simulink model "gm_uz_ssi_interface_2025b"  (R2025b)
settings: Solver=FixedStepDiscrete  StartTime=0.0  StopTime=0.005  RelTol=1e-3
undefined symbols (not defined in the file or in its folder): binary_or_gray, bit_sum, delay_first_clk_on_off, f_ADC, f_clock, PLL, ssi_clk_divider, ssi_encoder_bit_width_multi_turn, ssi_encoder_bit_width_single_turn, ssi_encoder_number_of_status_bits, t_ADC, t_clock, XData
libraries: hdlmdlgenlib x104, hdlsllib x90, simulink x33, simulink_extras x7
(part 4 of 4)

== system gm_uz_ssi_interface_2025b/uz_ssi_interface/position_to_speed_pll/Sine HDL Optimized1/sincos hdl ==
  In1 : Inport  OutDataTypeStr=fixdt(1, 27, 20)  SampleTime=1e-08
  cos_hdl : Subsystem  mask{NumDataPoints=double(256), TableDataTypeStr=fixdt(0,26,20), SimulateLUTROMDelay=Off}
      mask prompts: NumDataPoints "HDLShared:hdlshared:CosineHDL_Npts"; TableDataTypeStr "Simulink:blkprm_prompts:TABLE_UNIFIEDDATATYPE"; SimulateLUTROMDelay "HDLShared:hdlshared:CosineHDL_SimulateLUTDelay"
      mask init:
      | InputWordLength = double(10);
      | NumDataPoints = double(256);
      | OutputFracLength = double(20);
      | OutputWordLength = double(27);
      | SampleTime = double(-1);
      | SimulateLUTROMDelay = double(0);
      | TableDataTypeStr = fixdt(0,26,20);
      | TableFracLength = double(20);
      | TableWordLength = double(26);
      | YData = reshape(double([0;0.0061358846491544753;0.012271538285719925;0.01840672990580482;0.024541228522912288;0.030674803176636626;0.036807222941358832;0.04293825693494082;0.049067674327418015;0.055195244349689941;0.061320736302208578;0.067443919563664051;0.073564563599667426;0.079682437971430126;0.085797312344439894;0.091908956497132724;0.098017140329560604;0.10412163387205459;0.11022220729388306;0.11631863091190475;0.1224106751992162;0.12849811079379317;0.13458070850712617;0.14065823933284921;0.14673047445536175;0.15279718525844344;0.15885814333386145;0.16491312048996992;0.17096188876030122;0.17700422041214875;0.18303988795514095;0.18906866414980619;0.19509032201612825;0.2011046348420919;0.20711137619221856;0.21311031991609136;0.2191012401568698;0.22508391135979283;0.23105810828067111;0.2370236059943672;0.24298017990326387;0.24892760574572015;0.25486565960451457;0.26079411791527551;0.26671275747489837;0.27262135544994898;0.27851968938505306;0.28440753721127188;0.29028467725446233;0.29615088824362379;0.30200594931922808;0.30784964004153487;0.31368174039889152;0.31950203081601569;0.32531029216226293;0.33110630575987643;0.33688985339222005;0.34266071731199438;0.34841868024943456;0.35416352542049034;0.35989503653498811;0.36561299780477385;0.37131719395183749;0.37700741021641826;0.38268343236508978;0.38834504669882625;0.3939920400610481;0.39962419984564679;0.40524131400498986;0.41084317105790391;0.41642956009763715;0.42200027079979968;0.42755509343028208;0.43309381885315196;0.43861623853852766;0.4441221445704292;0.44961132965460654;0.45508358712634384;0.46053871095824001;0.46597649576796618;0.47139673682599764;0.47679923006332209;0.48218377207912272;0.487550160148436;0.49289819222978404;0.49822766697278181;0.50353838372571758;0.50883014254310699;0.51410274419322166;0.51935599016558964;0.52458968267846895;0.52980362468629461;0.53499761988709715;0.54017147272989285;0.54532498842204646;0.55045797293660481;0.55557023301960218;0.56066157619733603;0.56573181078361312;0.57078074588696726;0.57580819141784534;0.58081395809576453;0.58579785745643886;0.59075970185887416;0.59569930449243336;0.60061647938386897;0.60551104140432555;0.61038280627630948;0.61523159058062682;0.6200572117632891;0.62485948814238634;0.62963823891492698;0.63439328416364549;0.63912444486377573;0.64383154288979139;0.64851440102211244;0.65317284295377676;0.65780669329707864;0.66241577759017178;0.66699992230363747;0.67155895484701833;0.67609270357531592;0.68060099779545302;0.68508366777270036;0.68954054473706683;0.69397146088965389;0.69837624940897292;0.7027547444572253;0.70710678118654746;0.71143219574521643;0.71573082528381859;0.72000250796138165;0.72424708295146689;0.7284643904482252;0.73265427167241282;0.73681656887736979;0.74095112535495911;0.74505778544146595;0.74913639452345926;0.75318679904361252;0.75720884650648457;0.76120238548426178;0.76516726562245896;0.76910333764557959;0.77301045336273688;0.77688846567323244;0.78073722857209438;0.78455659715557524;0.78834642762660623;0.79210657730021228;0.79583690460888357;0.79953726910790501;0.80320753148064483;0.80684755354379922;0.81045719825259477;0.8140363297059483;0.81758481315158371;0.82110251499110465;0.82458930278502529;0.8280450452577558;0.83146961230254524;0.83486287498638001;0.83822470555483797;0.84155497743689833;0.84485356524970701;0.84812034480329712;0.8513551931052652;0.85455798836540053;0.85772861000027212;0.86086693863776731;0.8639728561215867;0.86704624551569265;0.87008699110871135;0.87309497841829009;0.8760700941954066;0.87901222642863341;0.88192126434835494;0.88479709843093779;0.88763962040285393;0.89044872324475788;0.89322430119551532;0.89596624975618511;0.89867446569395382;0.90134884704602203;0.90398929312344334;0.90659570451491533;0.90916798309052238;0.91170603200542988;0.91420975570353069;0.9166790599210427;0.91911385169005777;0.9215140393420419;0.92387953251128674;0.92621024213831138;0.92850608047321559;0.93076696107898371;0.93299279883473885;0.9351835099389475;0.93733901191257496;0.93945922360218992;0.94154406518302081;0.94359345816196039;0.94560732538052128;0.94758559101774109;0.94952818059303667;0.95143502096900834;0.95330604035419375;0.95514116830577067;0.95694033573220894;0.9587034748958716;0.96043051941556579;0.96212140426904158;0.96377606579543984;0.9653944416976894;0.96697647104485207;0.96852209427441727;0.97003125319454397;0.97150389098625178;0.97293995220556007;0.97433938278557586;0.97570213003852857;0.97702814265775439;0.97831737071962765;0.97956976568544052;0.98078528040323043;0.98196386910955524;0.98310548743121629;0.98421009238692903;0.98527764238894122;0.98630809724459867;0.98730141815785843;0.98825756773074946;0.98917650996478101;0.99005821026229712;0.99090263542778001;0.99170975366909953;0.99247953459870997;0.9932119492347945;0.99390697000235606;0.99456457073425542;0.99518472667219682;0.99576741446765982;0.996312612182778;0.99682029929116567;0.99729045667869021;0.99772306664419164;0.99811811290014918;0.99847558057329477;0.99879545620517241;0.99907772775264536;0.99932238458834954;0.99952941750109314;0.99969881869620425;0.9998305817958234;0.9999247018391445;0.99998117528260111]), [1  256]);
      | block_name = 'uz_ssi_interface_2025b/uz_ssi_interface/position_to_speed_pll/Sine\nHDL Optimized1/sincos hdl/cos_hdl';
      | gcb_lut = double(11088.000122070312);
      mask Display:
      | port_label('input',1,'u')
      | port_label('output',1,'cos(2*pi*u)')
      | xpos = 0.35;
      | yoffset = 0.5;
      | if ( SimulateLUTROMDelay )
      |   text(xpos,yoffset,'HDL (Z^{-1})','texmode','on')
      | else
      |    text(xpos,yoffset,'HDL')
      | end
  sin_hdl : Subsystem  mask{NumDataPoints=double(256), TableDataTypeStr=fixdt(0,26,20), SimulateLUTROMDelay=Off}
      mask prompts: NumDataPoints "HDLShared:hdlshared:CosineHDL_Npts"; TableDataTypeStr "Simulink:blkprm_prompts:TABLE_UNIFIEDDATATYPE"; SimulateLUTROMDelay "HDLShared:hdlshared:CosineHDL_SimulateLUTDelay"
      mask init:
      | InputWordLength = double(10);
      | NumDataPoints = double(256);
      | OutputFracLength = double(20);
      | OutputWordLength = double(27);
      | SampleTime = double(-1);
      | SimulateLUTROMDelay = double(0);
      | TableDataTypeStr = fixdt(0,26,20);
      | TableFracLength = double(20);
      | TableWordLength = double(26);
      | YData = reshape(double([0;0.0061358846491544753;0.012271538285719925;0.01840672990580482;0.024541228522912288;0.030674803176636626;0.036807222941358832;0.04293825693494082;0.049067674327418015;0.055195244349689941;0.061320736302208578;0.067443919563664051;0.073564563599667426;0.079682437971430126;0.085797312344439894;0.091908956497132724;0.098017140329560604;0.10412163387205459;0.11022220729388306;0.11631863091190475;0.1224106751992162;0.12849811079379317;0.13458070850712617;0.14065823933284921;0.14673047445536175;0.15279718525844344;0.15885814333386145;0.16491312048996992;0.17096188876030122;0.17700422041214875;0.18303988795514095;0.18906866414980619;0.19509032201612825;0.2011046348420919;0.20711137619221856;0.21311031991609136;0.2191012401568698;0.22508391135979283;0.23105810828067111;0.2370236059943672;0.24298017990326387;0.24892760574572015;0.25486565960451457;0.26079411791527551;0.26671275747489837;0.27262135544994898;0.27851968938505306;0.28440753721127188;0.29028467725446233;0.29615088824362379;0.30200594931922808;0.30784964004153487;0.31368174039889152;0.31950203081601569;0.32531029216226293;0.33110630575987643;0.33688985339222005;0.34266071731199438;0.34841868024943456;0.35416352542049034;0.35989503653498811;0.36561299780477385;0.37131719395183749;0.37700741021641826;0.38268343236508978;0.38834504669882625;0.3939920400610481;0.39962419984564679;0.40524131400498986;0.41084317105790391;0.41642956009763715;0.42200027079979968;0.42755509343028208;0.43309381885315196;0.43861623853852766;0.4441221445704292;0.44961132965460654;0.45508358712634384;0.46053871095824001;0.46597649576796618;0.47139673682599764;0.47679923006332209;0.48218377207912272;0.487550160148436;0.49289819222978404;0.49822766697278181;0.50353838372571758;0.50883014254310699;0.51410274419322166;0.51935599016558964;0.52458968267846895;0.52980362468629461;0.53499761988709715;0.54017147272989285;0.54532498842204646;0.55045797293660481;0.55557023301960218;0.56066157619733603;0.56573181078361312;0.57078074588696726;0.57580819141784534;0.58081395809576453;0.58579785745643886;0.59075970185887416;0.59569930449243336;0.60061647938386897;0.60551104140432555;0.61038280627630948;0.61523159058062682;0.6200572117632891;0.62485948814238634;0.62963823891492698;0.63439328416364549;0.63912444486377573;0.64383154288979139;0.64851440102211244;0.65317284295377676;0.65780669329707864;0.66241577759017178;0.66699992230363747;0.67155895484701833;0.67609270357531592;0.68060099779545302;0.68508366777270036;0.68954054473706683;0.69397146088965389;0.69837624940897292;0.7027547444572253;0.70710678118654746;0.71143219574521643;0.71573082528381859;0.72000250796138165;0.72424708295146689;0.7284643904482252;0.73265427167241282;0.73681656887736979;0.74095112535495911;0.74505778544146595;0.74913639452345926;0.75318679904361252;0.75720884650648457;0.76120238548426178;0.76516726562245896;0.76910333764557959;0.77301045336273688;0.77688846567323244;0.78073722857209438;0.78455659715557524;0.78834642762660623;0.79210657730021228;0.79583690460888357;0.79953726910790501;0.80320753148064483;0.80684755354379922;0.81045719825259477;0.8140363297059483;0.81758481315158371;0.82110251499110465;0.82458930278502529;0.8280450452577558;0.83146961230254524;0.83486287498638001;0.83822470555483797;0.84155497743689833;0.84485356524970701;0.84812034480329712;0.8513551931052652;0.85455798836540053;0.85772861000027212;0.86086693863776731;0.8639728561215867;0.86704624551569265;0.87008699110871135;0.87309497841829009;0.8760700941954066;0.87901222642863341;0.88192126434835494;0.88479709843093779;0.88763962040285393;0.89044872324475788;0.89322430119551532;0.89596624975618511;0.89867446569395382;0.90134884704602203;0.90398929312344334;0.90659570451491533;0.90916798309052238;0.91170603200542988;0.91420975570353069;0.9166790599210427;0.91911385169005777;0.9215140393420419;0.92387953251128674;0.92621024213831138;0.92850608047321559;0.93076696107898371;0.93299279883473885;0.9351835099389475;0.93733901191257496;0.93945922360218992;0.94154406518302081;0.94359345816196039;0.94560732538052128;0.94758559101774109;0.94952818059303667;0.95143502096900834;0.95330604035419375;0.95514116830577067;0.95694033573220894;0.9587034748958716;0.96043051941556579;0.96212140426904158;0.96377606579543984;0.9653944416976894;0.96697647104485207;0.96852209427441727;0.97003125319454397;0.97150389098625178;0.97293995220556007;0.97433938278557586;0.97570213003852857;0.97702814265775439;0.97831737071962765;0.97956976568544052;0.98078528040323043;0.98196386910955524;0.98310548743121629;0.98421009238692903;0.98527764238894122;0.98630809724459867;0.98730141815785843;0.98825756773074946;0.98917650996478101;0.99005821026229712;0.99090263542778001;0.99170975366909953;0.99247953459870997;0.9932119492347945;0.99390697000235606;0.99456457073425542;0.99518472667219682;0.99576741446765982;0.996312612182778;0.99682029929116567;0.99729045667869021;0.99772306664419164;0.99811811290014918;0.99847558057329477;0.99879545620517241;0.99907772775264536;0.99932238458834954;0.99952941750109314;0.99969881869620425;0.9998305817958234;0.9999247018391445;0.99998117528260111]), [1  256]);
      | block_name = 'uz_ssi_interface_2025b/uz_ssi_interface/position_to_speed_pll/Sine\nHDL Optimized1/sincos hdl/sin_hdl';
      | gcb_lut = double(11232.000122070312);
      mask Display:
      | port_label('input',1,'u')
      | port_label('output',1,'sin(2*pi*u)')
      | xpos = 0.35;
      | yoffset = 0.5;
      | if ( SimulateLUTROMDelay )
      |   text(xpos,yoffset,'HDL (Z^{-1})','texmode','on')
      | else
      |    text(xpos,yoffset,'HDL')
      | end
  Out1 : Outport  SampleTime=1e-08  VectorParamsAs1DForOutWhenUnconnected=off
  Out2 : Outport  Port=2  SampleTime=1e-08  VectorParamsAs1DForOutWhenUnconnected=off
  wires:
  In1/1 -> cos_hdl/1(In1), sin_hdl/1(In1)
  sin_hdl/1(y) -> Out1/1
  cos_hdl/1(x) -> Out2/1

== system gm_uz_ssi_interface_2025b/uz_ssi_interface/ssi_communication/sample_serial_ssi_data/Sample and Hold1 ==
  In : Inport  OutDataTypeStr=boolean  SampleTime=1e-08
  S : Inport  Port=2  OutDataTypeStr=boolean  SampleTime=1e-08
  Model : Subsystem
  "   " : Outport  SampleTime=1e-08  InitialOutput=0  VectorParamsAs1DForOutWhenUnconnected=off
  wires:
  In/1 -> Model/1(In)
  S/1 -> Model/2(S)
  Model/1(Out) -> "   "/1

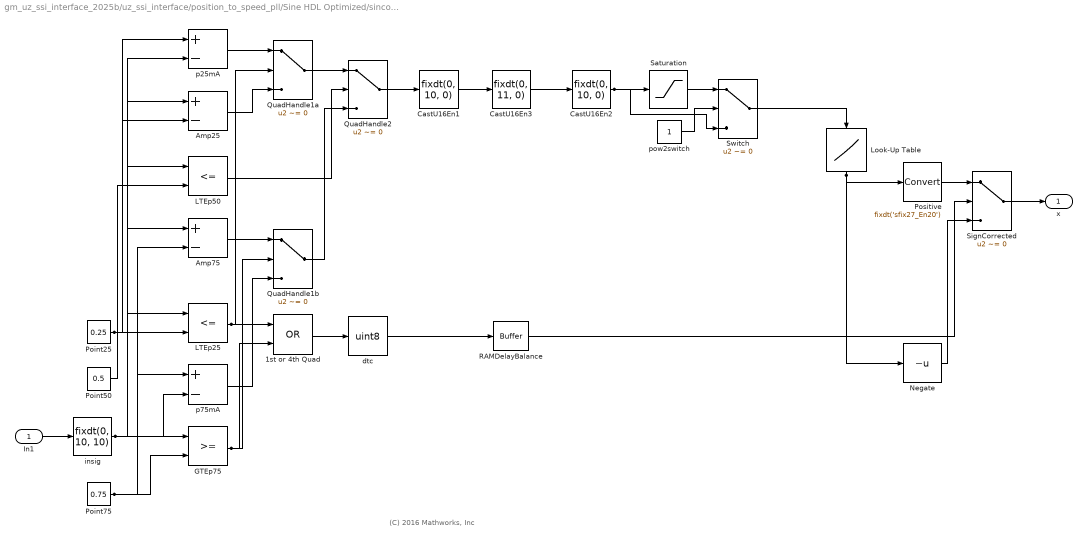
== system gm_uz_ssi_interface_2025b/uz_ssi_interface/position_to_speed_pll/Sine HDL Optimized/sincos hdl/cos_hdl ==
  note: (C) 2016 Mathworks, Inc
  In1 : Inport  OutDataTypeStr=fixdt(1, 27, 20)  SampleTime=1e-08
  1st or 4th Quad : Logic  Operator=OR  AllPortsSameDT=off  OutDataTypeStr=boolean  SampleTime=1e-08
  Amp25 : Sum  Inputs=+-  OutDataTypeStr=fixdt(1, 28, 27)  AccumDataTypeStr=fixdt(1, 28, 27)  SampleTime=1e-08
  Amp75 : Sum  Inputs=+-  OutDataTypeStr=fixdt(1, 28, 27)  AccumDataTypeStr=fixdt(1, 28, 27)  SampleTime=1e-08
  CastU16En1 : DataTypeConversion  OutDataTypeStr=fixdt(0, 10, 0)  ConvertRealWorld=Stored Integer (SI)  SampleTime=1e-08  SaturateOnIntegerOverflow=off  RndMeth=Floor
  CastU16En2 : DataTypeConversion  OutDataTypeStr=fixdt(0, 10, 0)  ConvertRealWorld=Stored Integer (SI)  SampleTime=1e-08  RndMeth=Floor
  CastU16En3 : DataTypeConversion  OutDataTypeStr=fixdt(0, 11, 0)  SampleTime=1e-08  SaturateOnIntegerOverflow=off  RndMeth=Floor
  GTEp75 : RelationalOperator  OutDataTypeStr=boolean  SampleTime=1e-08  InputSameDT=off
  LTEp25 : RelationalOperator  Operator=<=  OutDataTypeStr=boolean  SampleTime=1e-08  InputSameDT=off
  LTEp50 : RelationalOperator  Operator=<=  OutDataTypeStr=boolean  SampleTime=1e-08  InputSameDT=off
  Look-Up Table : Lookup_n-D  NumberOfTableDimensions=1  LookupTableObject=''  BreakpointsSpecification=Even spacing  BreakpointsForDimension1=XData  BreakpointsForDimension1FirstPoint=fi(0,0,InputWordLength,0)  BreakpointsForDimension1Spacing=fi(1,0,InputWordLength,0)  IndexSearchMethod=Evenly spaced points  Table=fi(YData,0, TableWordLength, TableFracLength)  TableDataTypeStr=fixdt(0, TableWordLength, TableFracLength)  InterpMethod=Flat  ExtrapMethod=Clip  OutDataTypeStr=fixdt(1,OutputWordLength,OutputFracLength)  LockScale=on
  Negate : UnaryMinus  SampleTime=1e-08
  Point25 : Constant  Value=0.25  OutDataTypeStr=fixdt(0, 27, 27)  SampleTime=1e-08
  Point50 : Constant  Value=0.5  OutDataTypeStr=fixdt(0, 27, 27)  SampleTime=1e-08
  Point75 : Constant  Value=0.75  OutDataTypeStr=fixdt(0, 27, 27)  SampleTime=1e-08
  Positive : DataTypeConversion  OutDataTypeStr=fixdt('sfix27_En20')
  QuadHandle1a : Switch  Criteria=u2 ~= 0  Threshold="fi(0,0,1,0,\"hex\",\"0\")"  OutDataTypeStr=fixdt(1, 28, 27)  SampleTime=1e-08  SaturateOnIntegerOverflow=off  InputSameDT=off
  QuadHandle1b : Switch  Criteria=u2 ~= 0  Threshold="fi(0,0,1,0,\"hex\",\"0\")"  OutDataTypeStr=fixdt(1, 28, 27)  SampleTime=1e-08  SaturateOnIntegerOverflow=off  InputSameDT=off
  QuadHandle2 : Switch  Criteria=u2 ~= 0  Threshold="fi(0,0,1,0,\"hex\",\"0\")"  OutDataTypeStr=fixdt(0, 10, 10)  SampleTime=1e-08  InputSameDT=off
  RAMDelayBalance : hdlmdlgenlib/Buffer
  Saturation : Saturate  UpperLimit="fi(0,0,10,0,\"hex\",\"0ff\")"  LowerLimit="fi(0,0,10,0,\"hex\",\"000\")"  SampleTime=1e-08  OutDataTypeStr=fixdt(0, 10, 0)
  SignCorrected : Switch  Criteria=u2 ~= 0  Threshold="fi(0,0,8,0,\"hex\",\"00\")"  OutDataTypeStr=fixdt(1, 27, 20)  SampleTime=1e-08  SaturateOnIntegerOverflow=off  InputSameDT=off
  Switch : Switch  Criteria=u2 ~= 0  Threshold="fi(0,0,1,0,\"hex\",\"0\")"  OutDataTypeStr=fixdt(0, 10, 0)  SampleTime=1e-08  SaturateOnIntegerOverflow=off  InputSameDT=off
  dtc : DataTypeConversion  OutDataTypeStr=uint8  ConvertRealWorld=Stored Integer (SI)  SampleTime=1e-08  SaturateOnIntegerOverflow=off  RndMeth=Floor
  insig : DataTypeConversion  OutDataTypeStr=fixdt(0, 10, 10)  SampleTime=1e-08  SaturateOnIntegerOverflow=off  RndMeth=Floor
  p25mA : Sum  Inputs=+-  OutDataTypeStr=fixdt(1, 28, 27)  AccumDataTypeStr=fixdt(1, 28, 27)  SampleTime=1e-08
  p75mA : Sum  Inputs=+-  OutDataTypeStr=fixdt(1, 28, 27)  AccumDataTypeStr=fixdt(1, 28, 27)  SampleTime=1e-08
  pow2switch : Constant  OutDataTypeStr=boolean  SampleTime=1e-08
  x : Outport  SampleTime=1e-08  VectorParamsAs1DForOutWhenUnconnected=off
  wires:
  In1/1 -> insig/1
  p25mA/1 -> QuadHandle1a/1
  Point25/1 -> p25mA/1, LTEp25/2, Amp25/2
  Point50/1 -> LTEp50/2
  Amp25/1 -> QuadHandle1a/3
  insig/1 -> p25mA/2, LTEp50/1, LTEp25/1, GTEp75/1, Amp75/1, p75mA/2, Amp25/1
  Point75/1 -> GTEp75/2, p75mA/1, Amp75/2
  LTEp50/1 -> QuadHandle2/2
  Amp75/1 -> QuadHandle1b/1
  LTEp25/1 -> QuadHandle1a/2, 1st or 4th Quad/1
  p75mA/1 -> QuadHandle1b/3
  GTEp75/1 -> QuadHandle1b/2, 1st or 4th Quad/2
  QuadHandle1a/1 -> QuadHandle2/1
  QuadHandle1b/1 -> QuadHandle2/3
  1st or 4th Quad/1 -> dtc/1
  Saturation/1 -> Switch/1
  QuadHandle2/1 -> CastU16En1/1
  dtc/1 -> RAMDelayBalance/1
  CastU16En1/1 -> CastU16En3/1
  CastU16En2/1 -> Switch/3, Saturation/1
  CastU16En3/1 -> CastU16En2/1
  RAMDelayBalance/1 -> SignCorrected/2
  SignCorrected/1 -> x/1
  pow2switch/1 -> Switch/2
  Switch/1 -> Look-Up Table/1
  Look-Up Table/1 -> Positive/1, Negate/1
  Positive/1 -> SignCorrected/1
  Negate/1 -> SignCorrected/3

== system gm_uz_ssi_interface_2025b/uz_ssi_interface/position_to_speed_pll/Sine HDL Optimized/sincos hdl/sin_hdl ==
  note: (C) 2016 Mathworks, Inc
  In1 : Inport  OutDataTypeStr=fixdt(1, 27, 20)  SampleTime=1e-08
  Amp50 : Sum  Inputs=+-  OutDataTypeStr=fixdt(1, 28, 27)  AccumDataTypeStr=fixdt(1, 28, 27)  SampleTime=1e-08
  CastU16En2 : DataTypeConversion  OutDataTypeStr=fixdt(0, 10, 0)  ConvertRealWorld=Stored Integer (SI)  SampleTime=1e-08  SaturateOnIntegerOverflow=off  RndMeth=Floor
  CastU16En3 : DataTypeConversion  OutDataTypeStr=fixdt(0, 10, 0)  ConvertRealWorld=Stored Integer (SI)  SampleTime=1e-08  RndMeth=Floor
  CastU16En4 : DataTypeConversion  OutDataTypeStr=fixdt(0, 11, 0)  SampleTime=1e-08  SaturateOnIntegerOverflow=off  RndMeth=Floor
  LTEp25 : RelationalOperator  Operator=<=  OutDataTypeStr=boolean  SampleTime=1e-08  InputSameDT=off
  LTEp50 : RelationalOperator  Operator=<=  OutDataTypeStr=boolean  SampleTime=1e-08  InputSameDT=off
  Look-Up Table : Lookup_n-D  NumberOfTableDimensions=1  LookupTableObject=''  BreakpointsSpecification=Even spacing  BreakpointsForDimension1=XData  BreakpointsForDimension1FirstPoint=fi(0,0,InputWordLength,0)  BreakpointsForDimension1Spacing=fi(1,0,InputWordLength,0)  IndexSearchMethod=Evenly spaced points  Table=fi(YData,0, TableWordLength, TableFracLength)  TableDataTypeStr=fixdt(0, TableWordLength, TableFracLength)  InterpMethod=Flat  ExtrapMethod=Clip  OutDataTypeStr=fixdt(1,OutputWordLength,OutputFracLength)  LockScale=on
  Negate : UnaryMinus  SampleTime=1e-08
  Point25 : Constant  Value=0.25  OutDataTypeStr=fixdt(0, 27, 27)  SampleTime=1e-08
  Point50 : Constant  Value=0.5  OutDataTypeStr=fixdt(0, 27, 27)  SampleTime=1e-08
  Positive : DataTypeConversion  OutDataTypeStr=fixdt('sfix27_En20')
  QuadHandle1 : Switch  Criteria=u2 ~= 0  Threshold="fi(0,0,1,0,\"hex\",\"0\")"  OutDataTypeStr=fixdt(1, 28, 27)  SampleTime=1e-08  SaturateOnIntegerOverflow=off  InputSameDT=off
  QuadHandle2 : Switch  Criteria=u2 ~= 0  Threshold="fi(0,0,1,0,\"hex\",\"0\")"  OutDataTypeStr=fixdt(0, 10, 10)  SampleTime=1e-08  SaturateOnIntegerOverflow=off  InputSameDT=off
  RAMDelayBalance : hdlmdlgenlib/Buffer
  Saturation : Saturate  UpperLimit="fi(0,0,10,0,\"hex\",\"0ff\")"  LowerLimit="fi(0,0,10,0,\"hex\",\"000\")"  SampleTime=1e-08  OutDataTypeStr=fixdt(0, 10, 0)
  SignCorrected : Switch  Criteria=u2 ~= 0  Threshold="fi(0,0,1,0,\"hex\",\"0\")"  OutDataTypeStr=fixdt(1, 27, 20)  SampleTime=1e-08  SaturateOnIntegerOverflow=off  InputSameDT=off
  Switch : Switch  Criteria=u2 ~= 0  Threshold="fi(0,0,1,0,\"hex\",\"0\")"  OutDataTypeStr=fixdt(0, 10, 0)  SampleTime=1e-08  SaturateOnIntegerOverflow=off  InputSameDT=off
  insig : DataTypeConversion  OutDataTypeStr=fixdt(0, 10, 10)  SampleTime=1e-08  SaturateOnIntegerOverflow=off  RndMeth=Floor
  p50mA : Sum  Inputs=+-  OutDataTypeStr=fixdt(1, 29, 27)  AccumDataTypeStr=fixdt(1, 29, 27)  SampleTime=1e-08
  pow2switch : Constant  OutDataTypeStr=boolean  SampleTime=1e-08
  y : Outport  SampleTime=1e-08  VectorParamsAs1DForOutWhenUnconnected=off
  wires:
  LTEp25/1 -> QuadHandle2/2
  Negate/1 -> SignCorrected/3
  QuadHandle1/1 -> QuadHandle2/1, p50mA/2, LTEp25/1
  Point50/1 -> p50mA/1, LTEp50/2, Amp50/2
  In1/1 -> insig/1
  Switch/1 -> Look-Up Table/1
  insig/1 -> QuadHandle1/1, LTEp50/1, Amp50/1
  Amp50/1 -> QuadHandle1/3
  LTEp50/1 -> RAMDelayBalance/1, QuadHandle1/2
  Point25/1 -> LTEp25/2
  p50mA/1 -> QuadHandle2/3
  RAMDelayBalance/1 -> SignCorrected/2
  QuadHandle2/1 -> CastU16En2/1
  CastU16En3/1 -> Switch/3, Saturation/1
  CastU16En2/1 -> CastU16En4/1
  CastU16En4/1 -> CastU16En3/1
  Saturation/1 -> Switch/1
  pow2switch/1 -> Switch/2
  Look-Up Table/1 -> Positive/1, Negate/1
  Positive/1 -> SignCorrected/1
  SignCorrected/1 -> y/1

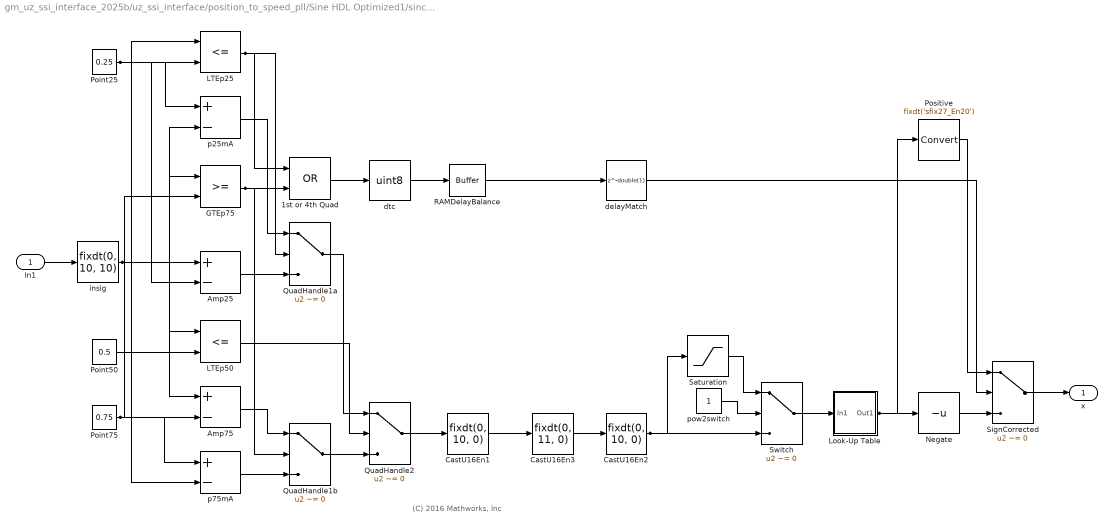
== system gm_uz_ssi_interface_2025b/uz_ssi_interface/position_to_speed_pll/Sine HDL Optimized1/sincos hdl/cos_hdl ==
  note: (C) 2016 Mathworks, Inc
  In1 : Inport  OutDataTypeStr=fixdt(1, 27, 20)  SampleTime=1e-08
  1st or 4th Quad : Logic  Operator=OR  AllPortsSameDT=off  OutDataTypeStr=boolean  SampleTime=1e-08
  Amp25 : Sum  Inputs=+-  OutDataTypeStr=fixdt(1, 28, 27)  AccumDataTypeStr=fixdt(1, 28, 27)  SampleTime=1e-08
  Amp75 : Sum  Inputs=+-  OutDataTypeStr=fixdt(1, 28, 27)  AccumDataTypeStr=fixdt(1, 28, 27)  SampleTime=1e-08
  CastU16En1 : DataTypeConversion  OutDataTypeStr=fixdt(0, 10, 0)  ConvertRealWorld=Stored Integer (SI)  SampleTime=1e-08  SaturateOnIntegerOverflow=off  RndMeth=Floor
  CastU16En2 : DataTypeConversion  OutDataTypeStr=fixdt(0, 10, 0)  ConvertRealWorld=Stored Integer (SI)  SampleTime=1e-08  RndMeth=Floor
  CastU16En3 : DataTypeConversion  OutDataTypeStr=fixdt(0, 11, 0)  SampleTime=1e-08  SaturateOnIntegerOverflow=off  RndMeth=Floor
  GTEp75 : RelationalOperator  OutDataTypeStr=boolean  SampleTime=1e-08  InputSameDT=off
  LTEp25 : RelationalOperator  Operator=<=  OutDataTypeStr=boolean  SampleTime=1e-08  InputSameDT=off
  LTEp50 : RelationalOperator  Operator=<=  OutDataTypeStr=boolean  SampleTime=1e-08  InputSameDT=off
  Look-Up Table : Subsystem
  Negate : UnaryMinus  SampleTime=1e-08
  Point25 : Constant  Value=0.25  OutDataTypeStr=fixdt(0, 27, 27)  SampleTime=1e-08
  Point50 : Constant  Value=0.5  OutDataTypeStr=fixdt(0, 27, 27)  SampleTime=1e-08
  Point75 : Constant  Value=0.75  OutDataTypeStr=fixdt(0, 27, 27)  SampleTime=1e-08
  Positive : DataTypeConversion  OutDataTypeStr=fixdt('sfix27_En20')
  QuadHandle1a : Switch  Criteria=u2 ~= 0  Threshold="fi(0,0,1,0,\"hex\",\"0\")"  OutDataTypeStr=fixdt(1, 28, 27)  SampleTime=1e-08  SaturateOnIntegerOverflow=off  InputSameDT=off
  QuadHandle1b : Switch  Criteria=u2 ~= 0  Threshold="fi(0,0,1,0,\"hex\",\"0\")"  OutDataTypeStr=fixdt(1, 28, 27)  SampleTime=1e-08  SaturateOnIntegerOverflow=off  InputSameDT=off
  QuadHandle2 : Switch  Criteria=u2 ~= 0  Threshold="fi(0,0,1,0,\"hex\",\"0\")"  OutDataTypeStr=fixdt(0, 10, 10)  SampleTime=1e-08  InputSameDT=off
  RAMDelayBalance : hdlmdlgenlib/Buffer
  Saturation : Saturate  UpperLimit="fi(0,0,10,0,\"hex\",\"0ff\")"  LowerLimit="fi(0,0,10,0,\"hex\",\"000\")"  SampleTime=1e-08  OutDataTypeStr=fixdt(0, 10, 0)
  SignCorrected : Switch  Criteria=u2 ~= 0  Threshold="fi(0,0,8,0,\"hex\",\"00\")"  OutDataTypeStr=fixdt(1, 27, 20)  SampleTime=1e-08  SaturateOnIntegerOverflow=off  InputSameDT=off
  Switch : Switch  Criteria=u2 ~= 0  Threshold="fi(0,0,1,0,\"hex\",\"0\")"  OutDataTypeStr=fixdt(0, 10, 0)  SampleTime=1e-08  SaturateOnIntegerOverflow=off  InputSameDT=off
  delayMatch : Delay  DelayLength=double(1)  InitialCondition=0
  dtc : DataTypeConversion  OutDataTypeStr=uint8  ConvertRealWorld=Stored Integer (SI)  SampleTime=1e-08  SaturateOnIntegerOverflow=off  RndMeth=Floor
  insig : DataTypeConversion  OutDataTypeStr=fixdt(0, 10, 10)  SampleTime=1e-08  SaturateOnIntegerOverflow=off  RndMeth=Floor
  p25mA : Sum  Inputs=+-  OutDataTypeStr=fixdt(1, 28, 27)  AccumDataTypeStr=fixdt(1, 28, 27)  SampleTime=1e-08
  p75mA : Sum  Inputs=+-  OutDataTypeStr=fixdt(1, 28, 27)  AccumDataTypeStr=fixdt(1, 28, 27)  SampleTime=1e-08
  pow2switch : Constant  OutDataTypeStr=boolean  SampleTime=1e-08
  x : Outport  SampleTime=1e-08  VectorParamsAs1DForOutWhenUnconnected=off
  wires:
  GTEp75/1 -> QuadHandle1b/2, 1st or 4th Quad/2
  In1/1 -> insig/1
  delayMatch/1 -> SignCorrected/2
  Point25/1 -> p25mA/1, LTEp25/2, Amp25/2
  Point50/1 -> LTEp50/2
  insig/1 -> p25mA/2, LTEp25/1, GTEp75/1, p75mA/2, Amp75/1, Amp25/1, LTEp50/1
  pow2switch/1 -> Switch/2
  QuadHandle1a/1 -> QuadHandle2/1
  Point75/1 -> GTEp75/2, Amp75/2, p75mA/1
  LTEp25/1 -> 1st or 4th Quad/1, QuadHandle1a/2
  p25mA/1 -> QuadHandle1a/1
  Amp25/1 -> QuadHandle1a/3
  LTEp50/1 -> QuadHandle2/2
  CastU16En1/1 -> CastU16En3/1
  Amp75/1 -> QuadHandle1b/1
  p75mA/1 -> QuadHandle1b/3
  1st or 4th Quad/1 -> dtc/1
  QuadHandle1b/1 -> QuadHandle2/3
  dtc/1 -> RAMDelayBalance/1
  QuadHandle2/1 -> CastU16En1/1
  RAMDelayBalance/1 -> delayMatch/1
  CastU16En3/1 -> CastU16En2/1
  CastU16En2/1 -> Switch/3, Saturation/1
  Saturation/1 -> Switch/1
  Switch/1 -> Look-Up Table/1(In1)
  Look-Up Table/1(Out1) -> Negate/1, Positive/1
  Negate/1 -> SignCorrected/3
  Positive/1 -> SignCorrected/1
  SignCorrected/1 -> x/1

== system gm_uz_ssi_interface_2025b/uz_ssi_interface/position_to_speed_pll/Sine HDL Optimized1/sincos hdl/sin_hdl ==
  note: (C) 2016 Mathworks, Inc
  In1 : Inport  OutDataTypeStr=fixdt(1, 27, 20)  SampleTime=1e-08
  Amp50 : Sum  Inputs=+-  OutDataTypeStr=fixdt(1, 28, 27)  AccumDataTypeStr=fixdt(1, 28, 27)  SampleTime=1e-08
  CastU16En2 : DataTypeConversion  OutDataTypeStr=fixdt(0, 10, 0)  ConvertRealWorld=Stored Integer (SI)  SampleTime=1e-08  SaturateOnIntegerOverflow=off  RndMeth=Floor
  CastU16En3 : DataTypeConversion  OutDataTypeStr=fixdt(0, 10, 0)  ConvertRealWorld=Stored Integer (SI)  SampleTime=1e-08  RndMeth=Floor
  CastU16En4 : DataTypeConversion  OutDataTypeStr=fixdt(0, 11, 0)  SampleTime=1e-08  SaturateOnIntegerOverflow=off  RndMeth=Floor
  LTEp25 : RelationalOperator  Operator=<=  OutDataTypeStr=boolean  SampleTime=1e-08  InputSameDT=off
  LTEp50 : RelationalOperator  Operator=<=  OutDataTypeStr=boolean  SampleTime=1e-08  InputSameDT=off
  Look-Up Table : Subsystem
  Negate : UnaryMinus  SampleTime=1e-08
  Point25 : Constant  Value=0.25  OutDataTypeStr=fixdt(0, 27, 27)  SampleTime=1e-08
  Point50 : Constant  Value=0.5  OutDataTypeStr=fixdt(0, 27, 27)  SampleTime=1e-08
  Positive : DataTypeConversion  OutDataTypeStr=fixdt('sfix27_En20')
  QuadHandle1 : Switch  Criteria=u2 ~= 0  Threshold="fi(0,0,1,0,\"hex\",\"0\")"  OutDataTypeStr=fixdt(1, 28, 27)  SampleTime=1e-08  SaturateOnIntegerOverflow=off  InputSameDT=off
  QuadHandle2 : Switch  Criteria=u2 ~= 0  Threshold="fi(0,0,1,0,\"hex\",\"0\")"  OutDataTypeStr=fixdt(0, 10, 10)  SampleTime=1e-08  SaturateOnIntegerOverflow=off  InputSameDT=off
  RAMDelayBalance : hdlmdlgenlib/Buffer
  Saturation : Saturate  UpperLimit="fi(0,0,10,0,\"hex\",\"0ff\")"  LowerLimit="fi(0,0,10,0,\"hex\",\"000\")"  SampleTime=1e-08  OutDataTypeStr=fixdt(0, 10, 0)
  SignCorrected : Switch  Criteria=u2 ~= 0  Threshold="fi(0,0,1,0,\"hex\",\"0\")"  OutDataTypeStr=fixdt(1, 27, 20)  SampleTime=1e-08  SaturateOnIntegerOverflow=off  InputSameDT=off
  Switch : Switch  Criteria=u2 ~= 0  Threshold="fi(0,0,1,0,\"hex\",\"0\")"  OutDataTypeStr=fixdt(0, 10, 0)  SampleTime=1e-08  SaturateOnIntegerOverflow=off  InputSameDT=off
  delayMatch : Delay  DelayLength=double(1)  InitialCondition=0
  insig : DataTypeConversion  OutDataTypeStr=fixdt(0, 10, 10)  SampleTime=1e-08  SaturateOnIntegerOverflow=off  RndMeth=Floor
  p50mA : Sum  Inputs=+-  OutDataTypeStr=fixdt(1, 29, 27)  AccumDataTypeStr=fixdt(1, 29, 27)  SampleTime=1e-08
  pow2switch : Constant  OutDataTypeStr=boolean  SampleTime=1e-08
  y : Outport  SampleTime=1e-08  VectorParamsAs1DForOutWhenUnconnected=off
  wires:
  LTEp50/1 -> QuadHandle1/2, RAMDelayBalance/1
  Point50/1 -> p50mA/1, Amp50/2, LTEp50/2
  In1/1 -> insig/1
  RAMDelayBalance/1 -> delayMatch/1
  insig/1 -> QuadHandle1/1, LTEp50/1, Amp50/1
  Point25/1 -> LTEp25/2
  Amp50/1 -> QuadHandle1/3
  QuadHandle1/1 -> QuadHandle2/1, p50mA/2, LTEp25/1
  LTEp25/1 -> QuadHandle2/2
  p50mA/1 -> QuadHandle2/3
  delayMatch/1 -> SignCorrected/2
  Saturation/1 -> Switch/1
  QuadHandle2/1 -> CastU16En2/1
  CastU16En2/1 -> CastU16En4/1
  CastU16En4/1 -> CastU16En3/1
  CastU16En3/1 -> Switch/3, Saturation/1
  pow2switch/1 -> Switch/2
  Switch/1 -> Look-Up Table/1(In1)
  Look-Up Table/1(Out1) -> Positive/1, Negate/1
  Positive/1 -> SignCorrected/1
  Negate/1 -> SignCorrected/3
  SignCorrected/1 -> y/1

== system gm_uz_ssi_interface_2025b/uz_ssi_interface/ssi_communication/sample_serial_ssi_data/Sample and Hold1/Model ==
  In : Inport  OutDataTypeStr=boolean  SampleTime=1e-08
  S : Inport  Port=2  OutDataTypeStr=boolean  SampleTime=1e-08
  Data Type Conversion : DataTypeConversion  OutDataTypeStr=boolean
  IC=ic : UnitDelay  SampleTime=1e-08
  Switch : Switch  Criteria=u2 ~= 0  Threshold="fi(0,0,1,0,\"hex\",\"0\")"  OutDataTypeStr=boolean  SampleTime=1e-08  InputSameDT=off
  Out : Outport  SampleTime=1e-08  InitialOutput=0
  wires:
  S/1 -> Data Type Conversion/1
  In/1 -> Switch/1
  Data Type Conversion/1 -> Switch/2
  IC=ic/1 -> Switch/3
  Switch/1 -> Out/1, IC=ic/1

== system gm_uz_ssi_interface_2025b/uz_ssi_interface/position_to_speed_pll/Sine HDL Optimized1/sincos hdl/cos_hdl/Look-Up Table ==
  In1 : Inport
  Look-Up Table : Lookup_n-D  NumberOfTableDimensions=1  LookupTableObject=''  BreakpointsSpecification=Even spacing  BreakpointsForDimension1=XData  BreakpointsForDimension1FirstPoint=fi(0,0,InputWordLength,0)  BreakpointsForDimension1Spacing=fi(1,0,InputWordLength,0)  IndexSearchMethod=Evenly spaced points  Table=fi(YData,0, TableWordLength, TableFracLength)  TableDataTypeStr=fixdt(0, TableWordLength, TableFracLength)  InterpMethod=Flat  ExtrapMethod=Clip  OutDataTypeStr=fixdt(1,OutputWordLength,OutputFracLength)  LockScale=on
  Look-Up Table_pd1 : Delay  DelayLength=1
  Out1 : Outport
  wires:
  Look-Up Table_pd1/1 -> Out1/1
  In1/1 -> Look-Up Table/1
  Look-Up Table/1 -> Look-Up Table_pd1/1

== system gm_uz_ssi_interface_2025b/uz_ssi_interface/position_to_speed_pll/Sine HDL Optimized1/sincos hdl/sin_hdl/Look-Up Table ==
  In1 : Inport
  Look-Up Table : Lookup_n-D  NumberOfTableDimensions=1  LookupTableObject=''  BreakpointsSpecification=Even spacing  BreakpointsForDimension1=XData  BreakpointsForDimension1FirstPoint=fi(0,0,InputWordLength,0)  BreakpointsForDimension1Spacing=fi(1,0,InputWordLength,0)  IndexSearchMethod=Evenly spaced points  Table=fi(YData,0, TableWordLength, TableFracLength)  TableDataTypeStr=fixdt(0, TableWordLength, TableFracLength)  InterpMethod=Flat  ExtrapMethod=Clip  OutDataTypeStr=fixdt(1,OutputWordLength,OutputFracLength)  LockScale=on
  Look-Up Table_pd1 : Delay  DelayLength=1
  Out1 : Outport
  wires:
  Look-Up Table/1 -> Look-Up Table_pd1/1
  In1/1 -> Look-Up Table/1
  Look-Up Table_pd1/1 -> Out1/1

== matlab function gm_uz_ssi_interface_2025b/uz_ssi_interface/wrap_2pi/fixed_point_floor/fixed_point_floor ==
  settings: fimath=fimath('RoundingMethod', 'Floor','OverflowAction', 'Wrap','ProductMode', 'FullPrecision', 'SumMode', 'FullPrecision')
  data: x input; y output
function y = fcn(x)
%#codegen
x_floor = bitsra(x, x.FractionLength);  % Shift right to remove fraction
x_floor = bitsll(x_floor, x.FractionLength);  % Shift left to restore scale

y = x_floor;

== matlab function gm_uz_ssi_interface_2025b/uz_ssi_interface/position_to_speed_pll/fixed_point_floor/fixed_point_floor ==
  settings: fimath=fimath('RoundingMethod', 'Floor','OverflowAction', 'Wrap','ProductMode', 'FullPrecision', 'SumMode', 'FullPrecision')
  data: x input; y output
function y = fcn(x)
%#codegen
x_floor = bitsra(x, x.FractionLength);  % Shift right to remove fraction
x_floor = bitsll(x_floor, x.FractionLength);  % Shift left to restore scale

y = x_floor;

== matlab function gm_uz_ssi_interface_2025b/ssi_encoder_RLS_ST14bit/MATLAB Function ==
  data: u input; y output
function y = BinaryToGray(u)
%#codegen

y = bitxor(u,(bitshift(u,-1)));

== matlab function gm_uz_ssi_interface_2025b/ssi_encoder_kuebler_MT12bit_ST13bit/MATLAB Function ==
  data: u input; y output
function y = BinaryToGray(u)
%#codegen

y = bitxor(u,(bitshift(u,-1)));
